simulink model "hybrid_lht_accumulator_backup"  (R2019b)
settings: Solver=FixedStepDiscrete  StartTime=0.0  StopTime=inf  FixedStep=1/bt.frequency  RelTol=1e-3
InitFcn:
  | ht_hybrid_setup;
StopFcn:
  | ht_hybrid_compare;
undefined symbols (not defined in the file or in its folder): bt, height, Ntheta, nTheta, width
libraries: hdlsllib x52, simulink x24, visionhdlutilities x2, dspsrcs4 x1, visionhdlio x1, lib_hybrid_ht_kernel x1, visionsources x1
(part 5 of 5)

== matlab function hybrid_lht_accumulator_backup/Hybrid LHT/Hybrid LHT Accumulator/Accumulator Control ==
  data: shift output; clear output; address output; sel output; read output; idx output; sof input; eof input; fvalid input; hStart output; hEnd output; vStart output; vEnd output; valid output; mode input; ready input; rhomax input; thetamax input; debug_state output; shiftmax input
function [shift, clear, address, sel, read, idx, hStart, hEnd, vStart, vEnd, valid, debug_state]  = acc_fsm(sof, eof, fvalid, mode, ready, rhomax, thetamax, shiftmax)

IDLE = fi(0, 0, 3, 0);
VOTE = fi(1, 0, 3, 0);
BACKPROP = fi(2, 0, 3, 0);
READ = fi(3, 0, 3, 0);
CLEAR = fi(7, 0 , 3, 0);

persistent rhocounter;

persistent thetacounter;

persistent shiftcounter;

persistent current_state;

if isempty(rhocounter)
    rhocounter = fi(0, 0, 32, 0);
end

if isempty(thetacounter)
    thetacounter = fi(0, 0, 32, 0);
end

if isempty(shiftcounter)
    shiftcounter = fi(0, 0, 6, 0);
end

if isempty(current_state)
    current_state = IDLE;
end

switch current_state
    case IDLE
        % Set Control Output
        clear = false;
        address = rhocounter;
        read = false;
        idx = thetacounter;
        shift = shiftcounter;
        
        % Set debug
        debug_state = current_state;
        
        % Set Video Output
        hStart = false;
        hEnd = false;
        vStart = false;
        vEnd = false;
        valid = false;
        
        % Set Variables
        rhocounter = fi(0, 0, 32, 0);
        thetacounter = fi(0, 0, 32, 0);
        shiftcounter = fi(0, 0, 6, 0);
        
        % Set next state
        if sof && fvalid
            sel = true;
            current_state = VOTE;
        else
            sel = false;
            current_state = IDLE;
        end
        
    case VOTE
        % Set Control Output
        clear = false;
        address = rhocounter;
        sel = true;
        read = false;
        idx = thetacounter;
        shift = shiftcounter;
        
        % Set debug
        debug_state = current_state;
        
        % Set Video Output
        hStart = false;
        hEnd = false;
        vStart = false;
        vEnd = false;
        valid = false;
        
        % Set Variables
        rhocounter = fi(0, 0, 32, 0);
        thetacounter = fi(0, 0, 32, 0);
        shiftcounter = fi(0, 0, 6, 0);
        
        % Set next state
        if eof && fvalid
            if mode
                current_state = BACKPROP;
            else
                current_state = READ;
            end
        else
            current_state = VOTE;
        end
         
    case BACKPROP
        % Set Control Output
        clear = true;
        address = rhocounter;
        sel = false;
        read = true;
        idx = thetacounter;
        shift = shiftcounter;
        
        % Set debug
        debug_state = current_state;
        
        shiftcounter = fi(0, 0, 6, 0);
        
        % Set Video Output
        hStart = false;
        hEnd = false;
        vStart = false;
        vEnd = false;
        valid = false;
        
        % Set next state
        if rhocounter >= rhomax
            current_state = IDLE;
        else
            % Set Variables
            rhocounter = fi(rhocounter + 1, 0, 32, 0);
            thetacounter = fi(0, 0, 32, 0);
            current_state = BACKPROP;
        end
        
    case READ
        % Set Control Output
        clear = false;
        address = rhocounter;
        sel = false;
        read = false;
        idx = thetacounter;
        shift = shiftcounter;
        
        % Set debug
        debug_state = current_state;
        
        % Set Video Output
        if rhocounter == 0
            hStart = true;
        else
            hStart = false;
        end
        
        if rhocounter == rhomax
            hEnd = true;
        else
            hEnd = false;
        end
        
        if rhocounter == 0 && thetacounter == 0 && shiftcounter == 0
            vStart = true;
        else
            vStart = false;
        end
        
        if rhocounter == rhomax && thetacounter == thetamax && shiftcounter == shiftmax
            vEnd = true;
        else
            vEnd = false;
        end
        
        if ready
            valid = true;
        else
            valid = false;
        end
        
        % Set next state
        if rhocounter >= rhomax && thetacounter >= thetamax && shiftcounter >= shiftmax
            rhocounter = fi(0, 0, 32, 0);
            thetacounter = fi(0, 0, 32, 0);
            shiftcounter = fi(0, 0, 6, 0);
            current_state = CLEAR;
        else
            if ready
                % Set Variables
                if thetacounter >= thetamax && rhocounter >= rhomax
                    rhocounter = fi(0, 0, 32, 0);
                    thetacounter = fi(0, 0, 32, 0);
                    shiftcounter = fi(shiftcounter + 1, 0, 6, 0);

                elseif rhocounter >= rhomax
                    rhocounter = fi(0, 0, 32, 0);
                    thetacounter = fi(thetacounter + 1, 0, 32, 0);

                else
                    rhocounter = fi(rhocounter + 1, 0, 32, 0);
                end
            end

            current_state = READ;
        end
        
    case CLEAR
        % Set Control Output
        clear = true;
        address = rhocounter;
        sel = false;
        read = false;
        idx = thetacounter;
        shift = shiftcounter;
        
        % Set debug
        debug_state = current_state;
        
        % Set Video Output
        hStart = false;
        hEnd = false;
        vStart = false;
        vEnd = false;
        valid = false;

        % Set next state
        if rhocounter >= rhomax
            current_state = IDLE;
        else
            % Set Variables
            rhocounter = fi(rhocounter + 1, 0, 32, 0);
            thetacounter = fi(0, 0, 32, 0);
            current_state = CLEAR;
        end
        
    otherwise
        % Set Control Output
        clear = false;
        address = rhocounter;
        sel = true;
        read = false;
        idx = thetacounter;
        shift = shiftcounter;
        
        % Set debug
        debug_state = current_state;
        
        % Set Video Output
        hStart = false;
        hEnd = false;
        vStart = false;
        vEnd = false;
        valid = false;
        
        % Set Variables
        rhocounter = fi(0, 0, 32, 0);
        thetacounter = fi(0, 0, 32, 0);
        
        % Set next state
        current_state = IDLE;
        
end
end
